simulink model "Mechanical_model_00"  (R2017a)
settings: Solver=VariableStepAuto  StartTime=0.0  StopTime=10.0  RelTol=1e-3
settings Model: Creator=uidn7735  LastModifiedBy=uidn7735

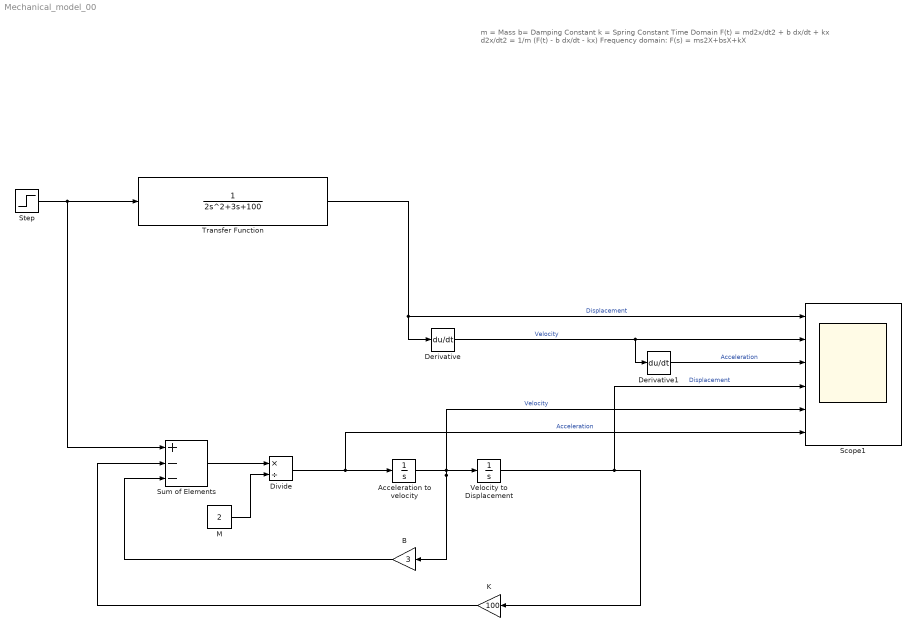
== system Mechanical_model_00 ==
  note: m = Mass
      |
      | b= Damping Constant
      |
      | k = Spring Constant
      |
      | Time Domain
      |
      | F(t) = md2x/dt2 + b dx/dt + kx
      |
      | d2x/dt2 = 1/m (F(t) - b dx/dt - kx)
      |
      | Frequency domain:
      |
      | F(s) = ms2X+bsX+kX
  Acceleration to velocity : Integrator
  B : Gain  Gain=3
  Derivative : Derivative
  Derivative1 : Derivative
  Divide : Product  Inputs=*/
  K : Gain  Gain=100
  M : Constant  Value=2
  Scope1 : Scope  NumInputPorts=6
  Step : Step  SampleTime=0
  Sum of Elements : Sum  Inputs=+--
  Transfer Function : TransferFcn  Denominator=[2 3 100]
  Velocity to Displacement : Integrator
  wires:
  Divide/1 -> Scope1/6, Acceleration to velocity/1  "Acceleration"
  K/1 -> Sum of Elements/2
  Sum of Elements/1 -> Divide/1
  Acceleration to velocity/1 -> Scope1/5, B/1, Velocity to Displacement/1  "Velocity"
  Step/1 -> Sum of Elements/1, Transfer Function/1
  M/1 -> Divide/2
  B/1 -> Sum of Elements/3
  Velocity to Displacement/1 -> Scope1/4, K/1  "Displacement"
  Transfer Function/1 -> Scope1/1, Derivative/1  "Displacement"
  Derivative/1 -> Scope1/2, Derivative1/1  "Velocity"
  Derivative1/1 -> Scope1/3  "Acceleration"
